simulink model "attack1"  (R2021a)
settings: Solver=FixedStepAuto  StartTime=0.0  StopTime=30  RelTol=1e-3
settings Model: Creator=Suman  LastModifiedBy=Suman

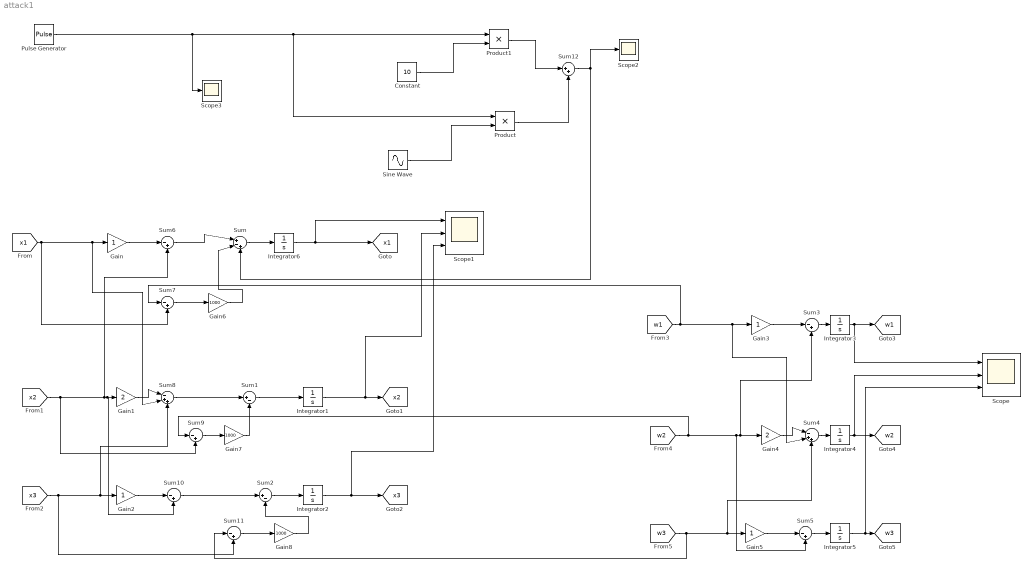
== system attack1 ==
  Constant : Constant  Value=10  SampleTime=0.001
  Gain{,2..3,5} (4 alike) : Gain
  Gain1 : Gain  Gain=2
  Gain4 : Gain  Gain=2
  Gain6 : Gain  Gain=1000
  Gain7 : Gain  Gain=1000
  Gain8 : Gain  Gain=1000
  Integrator1 : Integrator  InitialCondition=2
  Integrator2 : Integrator  InitialCondition=3
  Integrator3 : Integrator  InitialCondition=1
  Integrator4 : Integrator  InitialCondition=2
  Integrator5 : Integrator  InitialCondition=3
  Integrator6 : Integrator  InitialCondition=1
  Product : Product
  Product1 : Product
  Pulse Generator : DiscretePulseGenerator  PulseType=Time based  Period=30  PulseWidth=10  PhaseDelay=10
  Scope : Scope  NumInputPorts=3
  Scope1 : Scope  NumInputPorts=3
  Scope2 : Scope
  Scope3 : Scope
  Sine Wave : Sin  Amplitude=1000  SampleTime=0.001
  Sum : Sum  Inputs=|+-+
  Sum1 : Sum  Inputs=|+-
  Sum{3,5..7,9..11} (7 alike) : Sum  Inputs=|-+
  Sum12 : Sum  Inputs=|++
  Sum2 : Sum  Inputs=|+-
  Sum4 : Sum  Inputs=|-++
  Sum8 : Sum  Inputs=|-++
  tag scope: w1=global, w2=global, w3=global, x1=global, x2=global, x3=global
  wires:
  Gain3/1 -> Sum3/1
  Gain4/1 -> Sum4/1
  Sum3/1 -> Integrator3/1
  [w1] -> Sum4/2, Gain3/1, Sum7/1
  [w3] -> Gain5/1, Sum4/3, Sum11/1
  Gain5/1 -> Sum5/1
  [w2] -> Gain4/1, Sum3/2, Sum5/2, Sum9/1
  Sum4/1 -> Integrator4/1
  Sum5/1 -> Integrator5/1
  Gain/1 -> Sum6/1
  [x2] -> Sum10/2, Gain1/1, Sum6/2, Sum9/2
  Sum6/1 -> Sum/1
  Gain6/1 -> Sum/2
  Sum7/1 -> Gain6/1
  Sum/1 -> Integrator6/1
  Gain1/1 -> Sum8/1
  [x1] -> Sum8/2, Gain/1, Sum7/2
  [x3] -> Sum8/3, Gain2/1, Sum11/2
  Sum8/1 -> Sum1/1
  Sum1/1 -> Integrator1/1
  Sum9/1 -> Gain7/1
  Gain7/1 -> Sum1/2
  Gain2/1 -> Sum10/1
  Sum10/1 -> Sum2/1
  Sum2/1 -> Integrator2/1
  Sum11/1 -> Gain8/1
  Gain8/1 -> Sum2/2
  Constant/1 -> Product1/2
  Pulse Generator/1 -> Scope3/1, Product/1, Product1/1
  Product/1 -> Sum12/2
  Product1/1 -> Sum12/1
  Sum12/1 -> Sum/3, Scope2/1
  Sine Wave/1 -> Product/2
  Integrator3/1 -> Scope/1, [w1]
  Integrator4/1 -> Scope/2, [w2]
  Integrator5/1 -> Scope/3, [w3]
  Integrator6/1 -> Scope1/1, [x1]
  Integrator1/1 -> Scope1/2, [x2]
  Integrator2/1 -> Scope1/3, [x3]
